simulink model "Admittance"  (R2021a)
settings: Solver=VariableStepAuto  StartTime=0.0  StopTime=5  RelTol=1e-3
values from neighbouring files (symbols this model uses):
  kd = eye(6)*25    [params.m]
  KDt = 2*zt*wt    [params.m]
  kp = eye(6)*100    [params.m]
  KPt = wt^2    [params.m]
  Mt = 0.75*eye(6)    [params.m]
  x = [ 0.5357 ... (first row only)    [params.m]
settings Model: Creator=Sebastiano  LastModifiedBy=antoninoparisi
settings SolverCC: AlgebraicLoopSolver=TrustRegion
settings DebuggingCC: SFMachineParentedDataDiag=warning

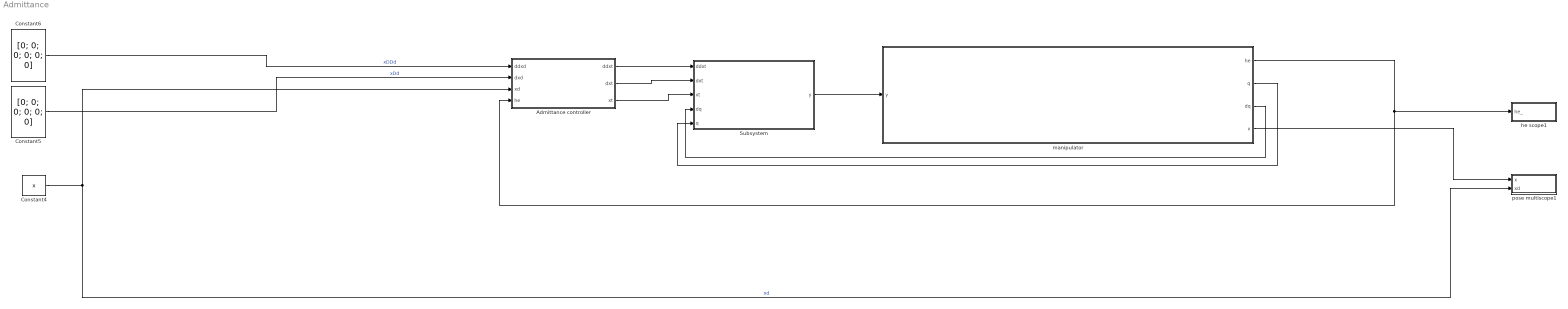
== system Admittance ==
  Admittance controller : Subsystem
  Constant4 : Constant  Value=x  VectorParams1D=off
  Constant5 : Constant  Value=[0; 0; 0; 0; 0; 0]  VectorParams1D=off
  Constant6 : Constant  Value=[0; 0; 0; 0; 0; 0]  VectorParams1D=off
  Subsystem : Subsystem
  he scope1 : Subsystem
  manipulator : Subsystem
  pose multiscope1 : Subsystem
  wires:
  manipulator/4(x) -> pose multiscope1/1(x)
  Constant4/1 -> Admittance controller/3(xd), pose multiscope1/2(xd)  "xd"
  Constant6/1 -> Admittance controller/1(ddxd)  "xDDd"
  Constant5/1 -> Admittance controller/2(dxd)  "xDd"
  manipulator/1(he) -> he scope1/1(he_), Admittance controller/4(he)
  manipulator/2(q) -> Subsystem/5(q)
  manipulator/3(dq) -> Subsystem/4(dq)
  Admittance controller/1(ddxt) -> Subsystem/1(ddxt)
  Admittance controller/2(dxt) -> Subsystem/2(dxt)
  Admittance controller/3(xt) -> Subsystem/3(xt)
  Subsystem/1(y) -> manipulator/1(y)

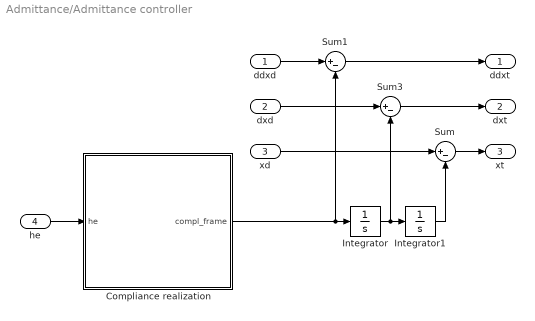
== system Admittance/Admittance controller ==
  ddxd : Inport
  dxd : Inport  Port=2
  xd : Inport  Port=3
  he : Inport  Port=4
  Compliance realization : Subsystem
  Integrator : Integrator
  Integrator1 : Integrator
  Sum : Sum  Inputs=|+-
  Sum1 : Sum  Inputs=|+-
  Sum3 : Sum  Inputs=|+-
  ddxt : Outport
  dxt : Outport  Port=2
  xt : Outport  Port=3
  wires:
  xd/1 -> Sum/1
  dxd/1 -> Sum3/1
  ddxd/1 -> Sum1/1
  Sum3/1 -> dxt/1
  Sum/1 -> xt/1
  Sum1/1 -> ddxt/1
  Integrator1/1 -> Sum/2
  Integrator/1 -> Sum3/2, Integrator1/1
  Compliance realization/1(compl_frame) -> Integrator/1, Sum1/2
  he/1 -> Compliance realization/1(he)

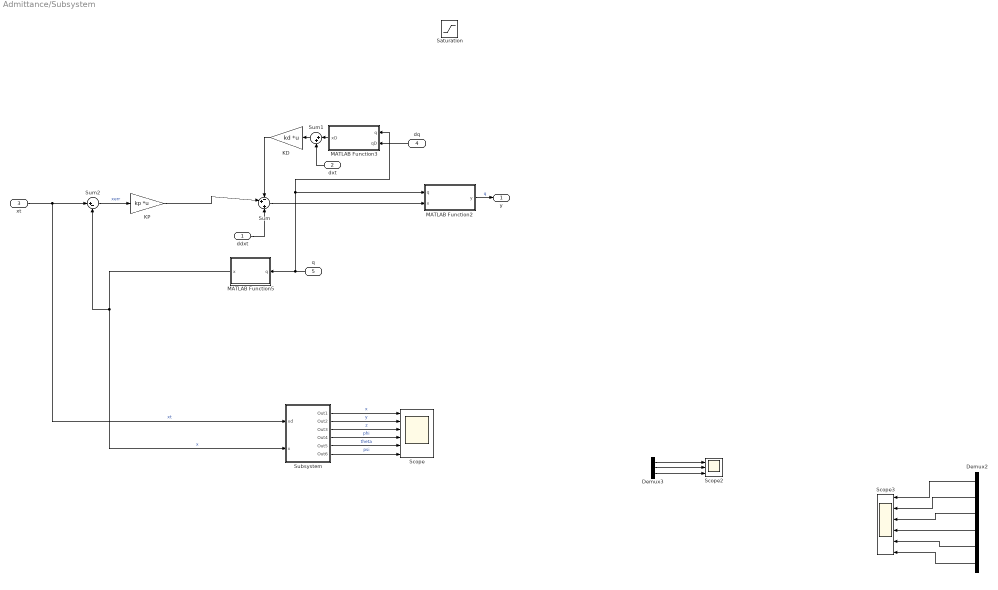
== system Admittance/Subsystem ==
  ddxt : Inport
  dxt : Inport  Port=2
  xt : Inport  Port=3
  dq : Inport  Port=4
  q : Inport  Port=5
  Demux2 : Demux  Outputs=6
  Demux3 : Demux  Outputs=3
  KD : Gain  Gain=kd  Multiplication=Matrix(K*u) (u vector)
  KP : Gain  Gain=kp  Multiplication=Matrix(K*u) (u vector)
  MATLAB Function2 : MATLAB Function  TreatAsAtomicUnit=on
  MATLAB Function3 : MATLAB Function  TreatAsAtomicUnit=on
  MATLAB Function5 : MATLAB Function  TreatAsAtomicUnit=on
  Saturation : Saturate  UpperLimit=500  LowerLimit=-500
  Scope : Scope  NumInputPorts=6
  Scope2 : Scope  NumInputPorts=3
  Scope3 : Scope  NumInputPorts=6
  Subsystem : Subsystem
  Sum : Sum  Inputs=-+|+
  Sum1 : Sum  Inputs=|++
  Sum2 : Sum  Inputs=|+-
  y : Outport
  wires:
  Demux2/3 -> Scope3/3
  Demux2/4 -> Scope3/4
  KP/1 -> Sum/2
  Subsystem/4(Out4) -> Scope/4  "phi"
  Demux2/6 -> Scope3/6
  Subsystem/1(Out1) -> Scope/1  "x"
  Demux3/3 -> Scope2/3
  Demux3/2 -> Scope2/2
  Sum/1 -> MATLAB Function2/2(x)
  Subsystem/6(Out6) -> Scope/6  "psi"
  MATLAB Function5/1(x) -> Subsystem/2(x), Sum2/2  "x"
  Subsystem/2(Out2) -> Scope/2  "y"
  KD/1 -> Sum/1
  Sum2/1 -> KP/1  "xerr"
  Subsystem/5(Out5) -> Scope/5  "theta"
  Demux2/5 -> Scope3/5
  Subsystem/3(Out3) -> Scope/3  "z"
  Demux3/1 -> Scope2/1
  xt/1 -> Subsystem/1(xd), Sum2/1  "xt"
  Demux2/1 -> Scope3/1
  Demux2/2 -> Scope3/2
  MATLAB Function2/1(y) -> y/1  "q"
  q/1 -> MATLAB Function3/1(q), MATLAB Function2/1(q), MATLAB Function5/1(q)
  dq/1 -> MATLAB Function3/2(qD)
  Sum1/1 -> KD/1
  MATLAB Function3/1(xD) -> Sum1/1
  dxt/1 -> Sum1/2
  ddxt/1 -> Sum/3

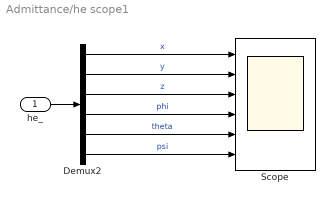
== system Admittance/he scope1 ==
  he_ : Inport
  Demux2 : Demux  Outputs=[1, 1, 1, 1, 1, 1]
  Scope : Scope  NumInputPorts=6
  wires:
  Demux2/4 -> Scope/4  "phi"
  Demux2/3 -> Scope/3  "z"
  Demux2/6 -> Scope/6  "psi"
  Demux2/5 -> Scope/5  "theta"
  Demux2/1 -> Scope/1  "x"
  he_/1 -> Demux2/1
  Demux2/2 -> Scope/2  "y"

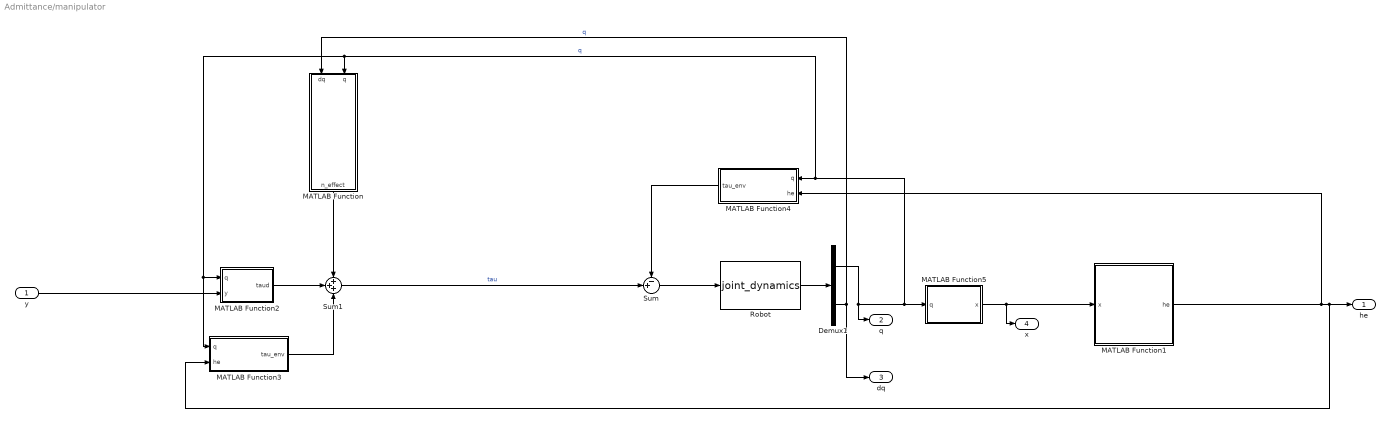
== system Admittance/manipulator ==
  y : Inport
  Demux1 : Demux  Outputs=[3, 3]
  MATLAB Function : MATLAB Function  TreatAsAtomicUnit=on
  MATLAB Function1 : MATLAB Function  TreatAsAtomicUnit=on
  MATLAB Function2 : MATLAB Function  TreatAsAtomicUnit=on
  MATLAB Function3 : MATLAB Function  TreatAsAtomicUnit=on
  MATLAB Function4 : MATLAB Function  TreatAsAtomicUnit=on
  MATLAB Function5 : MATLAB Function  TreatAsAtomicUnit=on
  Robot : S-Function  FunctionName=joint_dynamics  Parameters=robot  SFunctionDeploymentMode=off  EnableBusSupport=off
  Sum : Sum  Inputs=-+|
  Sum1 : Sum  Inputs=+++
  he : Outport
  q : Outport  Port=2
  dq : Outport  Port=3
  x : Outport  Port=4
  wires:
  Sum/1 -> Robot/1
  Robot/1 -> Demux1/1
  MATLAB Function4/1(tau_env) -> Sum/1
  MATLAB Function5/1(x) -> x/1, MATLAB Function1/1(x)
  MATLAB Function1/1(he) -> MATLAB Function4/2(he), MATLAB Function3/2(he), he/1
  Demux1/1 -> MATLAB Function5/1(q), MATLAB Function/2(q), MATLAB Function3/1(q), MATLAB Function2/1(q), MATLAB Function4/1(q), q/1  "q"
  y/1 -> MATLAB Function2/2(y)
  MATLAB Function/1(n_effect) -> Sum1/1
  Sum1/1 -> Sum/2  "tau"
  MATLAB Function3/1(tau_env) -> Sum1/3
  MATLAB Function2/1(taud) -> Sum1/2
  Demux1/2 -> dq/1, MATLAB Function/1(dq)  "q"

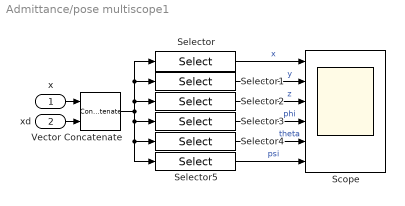
== system Admittance/pose multiscope1 ==
  x : Inport
  xd : Inport  Port=2
  Scope : Scope  NumInputPorts=6
  Selector : Selector  NumberOfDimensions=2  InputPortWidth=3  IndexOptions=Index vector (dialog),Select all  Indices=1,7  OutputSizes=6,6
  Selector1 : Selector  NumberOfDimensions=2  InputPortWidth=3  IndexOptions=Index vector (dialog),Select all  Indices=2,7  OutputSizes=6,6
  Selector2 : Selector  NumberOfDimensions=2  InputPortWidth=3  IndexOptions=Index vector (dialog),Select all  Indices=3,7  OutputSizes=6,6
  Selector3 : Selector  NumberOfDimensions=2  InputPortWidth=3  IndexOptions=Index vector (dialog),Select all  Indices=4,7  OutputSizes=6,6
  Selector4 : Selector  NumberOfDimensions=2  InputPortWidth=3  IndexOptions=Index vector (dialog),Select all  Indices=5,7  OutputSizes=6,6
  Selector5 : Selector  NumberOfDimensions=2  InputPortWidth=3  IndexOptions=Index vector (dialog),Select all  Indices=6,7  OutputSizes=6,6
  Vector Concatenate : Concatenate  Mode=Multidimensional array  ConcatenateDimension=2
  wires:
  x/1 -> Vector Concatenate/1
  xd/1 -> Vector Concatenate/2
  Selector1/1 -> Scope/2  "y"
  Selector5/1 -> Scope/6  "psi"
  Selector3/1 -> Scope/4  "phi"
  Selector/1 -> Scope/1  "x"
  Selector4/1 -> Scope/5  "theta"
  Vector Concatenate/1 -> Selector/1, Selector1/1, Selector2/1, Selector5/1, Selector4/1, Selector3/1
  Selector2/1 -> Scope/3  "z"

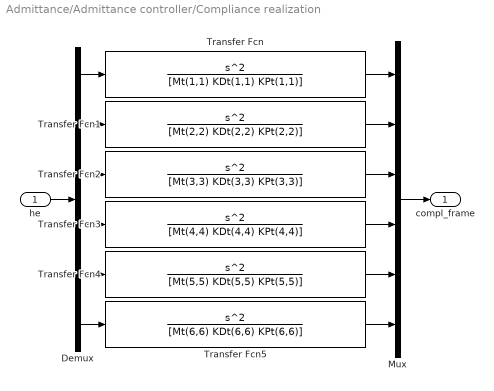
== system Admittance/Admittance controller/Compliance realization ==
  he : Inport
  Demux : Demux  Outputs=6
  Mux : Mux  Inputs=6
  Transfer Fcn : TransferFcn  Numerator=[1 0 0]  Denominator=[Mt(1,1) KDt(1,1) KPt(1,1)]
  Transfer Fcn1 : TransferFcn  Numerator=[1 0 0]  Denominator=[Mt(2,2) KDt(2,2) KPt(2,2)]
  Transfer Fcn2 : TransferFcn  Numerator=[1 0 0]  Denominator=[Mt(3,3) KDt(3,3) KPt(3,3)]
  Transfer Fcn3 : TransferFcn  Numerator=[1 0 0]  Denominator=[Mt(4,4) KDt(4,4) KPt(4,4)]
  Transfer Fcn4 : TransferFcn  Numerator=[1 0 0]  Denominator=[Mt(5,5) KDt(5,5) KPt(5,5)]
  Transfer Fcn5 : TransferFcn  Numerator=[1 0 0]  Denominator=[Mt(6,6) KDt(6,6) KPt(6,6)]
  compl_frame : Outport
  wires:
  Demux/5 -> Transfer Fcn4/1
  Transfer Fcn3/1 -> Mux/4
  Demux/4 -> Transfer Fcn3/1
  he/1 -> Demux/1
  Demux/1 -> Transfer Fcn/1
  Demux/6 -> Transfer Fcn5/1
  Transfer Fcn4/1 -> Mux/5
  Transfer Fcn2/1 -> Mux/3
  Mux/1 -> compl_frame/1
  Demux/2 -> Transfer Fcn1/1
  Transfer Fcn/1 -> Mux/1
  Demux/3 -> Transfer Fcn2/1
  Transfer Fcn5/1 -> Mux/6
  Transfer Fcn1/1 -> Mux/2

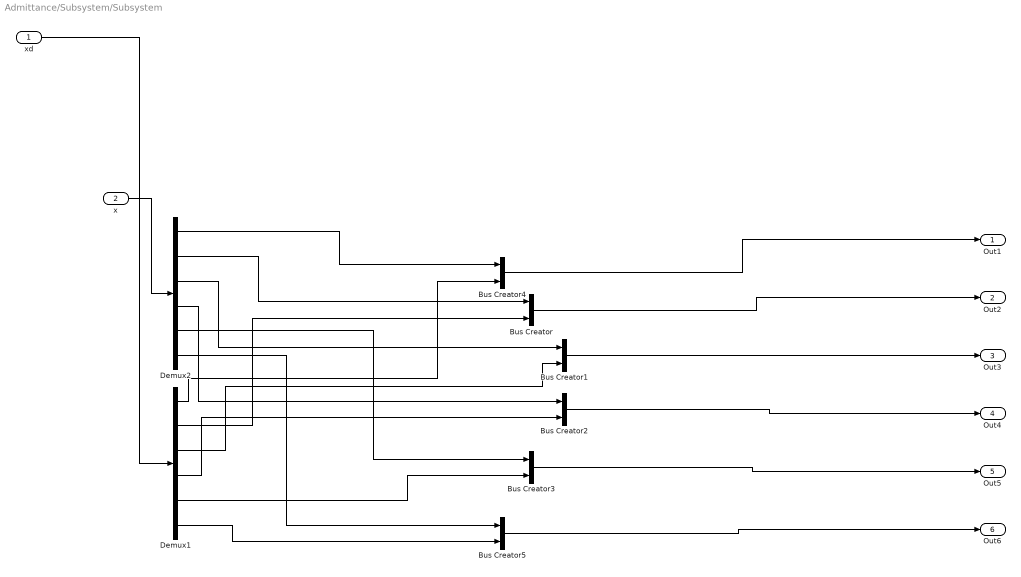
== system Admittance/Subsystem/Subsystem ==
  xd : Inport
  x : Inport  Port=2
  Bus Creator{,1..5} (6 alike) : BusCreator  Inputs=2
  Demux1 : Demux  Outputs=6
  Demux2 : Demux  Outputs=6
  Out1 : Outport
  Out2 : Outport  Port=2
  Out3 : Outport  Port=3
  Out4 : Outport  Port=4
  Out5 : Outport  Port=5
  Out6 : Outport  Port=6
  wires:
  xd/1 -> Demux1/1
  x/1 -> Demux2/1
  Bus Creator1/1 -> Out3/1
  Bus Creator4/1 -> Out1/1
  Demux2/2 -> Bus Creator/1
  Demux1/1 -> Bus Creator4/2
  Demux1/3 -> Bus Creator1/2
  Demux2/3 -> Bus Creator1/1
  Demux2/6 -> Bus Creator5/1
  Demux2/4 -> Bus Creator2/1
  Bus Creator5/1 -> Out6/1
  Demux2/1 -> Bus Creator4/1
  Bus Creator/1 -> Out2/1
  Demux1/6 -> Bus Creator5/2
  Demux1/2 -> Bus Creator/2
  Demux1/5 -> Bus Creator3/2
  Bus Creator2/1 -> Out4/1
  Demux1/4 -> Bus Creator2/2
  Bus Creator3/1 -> Out5/1
  Demux2/5 -> Bus Creator3/1

== matlab function Admittance/Subsystem/MATLAB Function2 ==
  data: q input; y output size=3; x input
function y = JAT(q, x)

y = analyticalJacobian(q)' * x;

== matlab function Admittance/Subsystem/MATLAB Function3 ==
  data: q input; xD output size=6; qD input
function xD = JA(q, qD)

xD = analyticalJacobian(q)*qD;

== matlab function Admittance/Subsystem/MATLAB Function5 ==
  data: q input; x output
function x = K(q)

t1 = q(1);
d1 = q(2);
t2 = q(3);


a1 = 0.15;
a2 = 0.4;
a3 = 0.3;
a4 = 0.16;


% wrt frame 0
K = [[cos(t1)*cos(t2), -cos(t1)*sin(t2), -sin(t1),      a2*cos(t1) + a4*cos(t1)*cos(t2)]
    [        sin(t2),          cos(t2),        0,                 a4*sin(t2) - d1 - a3]
    [cos(t2)*sin(t1), -sin(t1)*sin(t2),  cos(t1), a1 + a2*sin(t1) + a4*cos(t2)*sin(t1)]
    [              0,                0,        0,                                    1]];

pos = K(1:3, 4);
ori = rotm2eul(K(1:3,1:3), 'ZYZ')';

x = [pos; ori];

== matlab function Admittance/manipulator/MATLAB Function ==
  data: dq input; q input; n_effect output
function n_effect = n(dq, q)

n_effect = C_Lagrangian(q, dq)*dq + G_Lagrangian(q);

== matlab function Admittance/manipulator/MATLAB Function1 ==
  data: x input; he output
function he = environment(x)

% environment params
K = diag([2 2 2 0.1 0.1 0.1])*10;    % stiffness
wall = 0.16; % constraint position w.r.t. frame 0 (it's y=-0.5 w.r.t. base frame)

if abs(x(3)) >= wall  % check is done in frame 0
    % touching the environment! constrained motion
    % set up the rest position frame
    % (basically, same orientation as ee but position is the contact point at the wall)
    xr = x;
    xr(3) = wall;
    % calculate the forces
    dx_re = x - xr;
    he = K * dx_re;
else
    % free motion
    he = zeros(6,1);
end

he = reshape(he,[6 1]);

== matlab function Admittance/manipulator/MATLAB Function2 ==
  data: q input; taud output; y input
function taud = B(q, y)

taud = B_Lagrangian(q)*y;

== matlab function Admittance/manipulator/MATLAB Function3 ==
  data: q input; he input; tau_env output
function tau_env = J(q, he)

tau_env = jacobian(q)' * he;

== matlab function Admittance/manipulator/MATLAB Function4 ==
  data: q input; he input; tau_env output
function tau_env = J(q, he)

tau_env = jacobian(q)' * he;

== matlab function Admittance/manipulator/MATLAB Function5 ==
  data: q input; x output
function x = K(q)

t1 = q(1);
d1 = q(2);
t2 = q(3);


a1 = 0.15;
a2 = 0.4;
a3 = 0.3;
a4 = 0.16;


% wrt frame 0
K = [[cos(t1)*cos(t2), -cos(t1)*sin(t2), -sin(t1),      a2*cos(t1) + a4*cos(t1)*cos(t2)]
    [        sin(t2),          cos(t2),        0,                 a4*sin(t2) - d1 - a3]
    [cos(t2)*sin(t1), -sin(t1)*sin(t2),  cos(t1), a1 + a2*sin(t1) + a4*cos(t2)*sin(t1)]
    [              0,                0,        0,                                    1]];

pos = K(1:3, 4);
ori = rotm2eul(K(1:3,1:3), 'ZYZ')';

x = [pos; ori];
